simulink model "lyapunov_mras"  (R2019b)
settings: Solver=VariableStepAuto  StartTime=0.0  StopTime=50  RelTol=1e-3
values from neighbouring files (symbols this model uses):
  a = 2    [odev3.m]
  b = 1    [odev3.m]
  gamma1 = 4    [odev3.m]
  gamma2 = 0.2    [odev3.m]
settings Model: Creator=Mustafa Sezer  LastModifiedBy=Mustafa Sezer

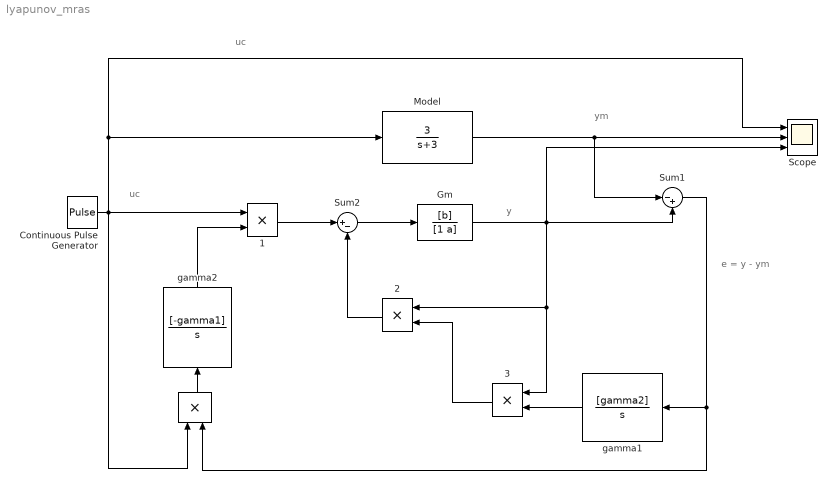
== system lyapunov_mras ==
  note: uc
  note: ym
  note: uc
  note: e = y - ym
  note: y
   {,1..3} (4 alike) : Product
  Continuous Pulse Generator : DiscretePulseGenerator  PulseType=Time based  Period=20  PulseWidth=50
  "Gm  " : TransferFcn  Numerator=[b]  Denominator=[1 a]
  Model : TransferFcn  Numerator=[3]  Denominator=[1 3]
  Scope : Scope  NumInputPorts=3
  Sum1 : Sum  Inputs=|-+
  Sum2 : Sum  Inputs=|+-
  gamma1 : TransferFcn  Numerator=[gamma2]  Denominator=[1 0]
  "gamma2 " : TransferFcn  Numerator=[-gamma1]  Denominator=[1 0]
  wires:
  Model/1 -> Scope/2, Sum1/1
  Continuous Pulse Generator/1 -> Model/1, Scope/1, " "/1, " 1"/1
  " "/1 -> "gamma2 "/1
  "gamma2 "/1 -> " 1"/2
  " 1"/1 -> Sum2/1
  Sum2/1 -> "Gm  "/1
  "Gm  "/1 -> " 2"/1, " 3"/1, Scope/3, Sum1/2
  Sum1/1 -> gamma1/1, " "/2
  gamma1/1 -> " 3"/2
  " 3"/1 -> " 2"/2
  " 2"/1 -> Sum2/2
